simulink model "DeltaWingPlantADRC_FINAL_2018a"  (Simulink 9.1)
settings: Solver=ode45  StartTime=0.0  StopTime=100  MaxStep=0.01  RelTol=1e-3  EnableMultiTasking=on
values from neighbouring files (symbols this model uses):
  beta0 = 0.4    [SA_ACex6_INIT.m]
  betap0 = 0    [SA_ACex6_INIT.m]
  Ta = 0.01    [SA_ACex6_INIT.m]
  um = pi    (= 3.14159265359)    [SA_ACex6_INIT.m]
libraries: simulink x1
settings Model: Creator=Adam  LastModifiedBy=Adam
settings DataIOCC: LimitDataPoints=on  SignalLoggingSaveFormat=ModelDataLogs
settings OptimizationCC: InitFltsAndDblsToZero=on
settings DebuggingCC: SaveWithParameterizedLinksMsg=none  SignalResolutionControl=TryResolveAllWithWarning  SolverPrmCheckMsg=warning  MultiTaskDSMMsg=warning  MultiTaskCondExecSysMsg=none  FcnCallInpInsideContextMsg=warning
settings SFSimCC: SimUseLocalCustomCode=on
settings RTWCC: RTWUseLocalCustomCode=on
settings GRTTargetCC: TargetFcnLib=ansi_tfl_tmw.mat
settings ConfigComp: CovExternalEMLEnable=on

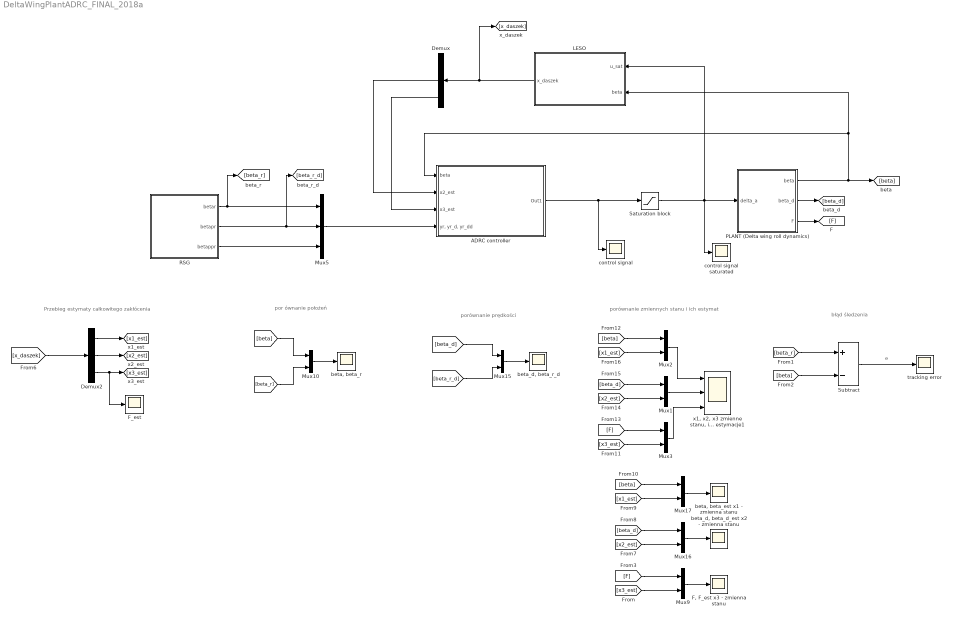
== system DeltaWingPlantADRC_FINAL_2018a ==
  note: Przebieg estymaty całkowitego zakłócenia
  note: błąd śledzenia
  note: e
  note: porównanie prędkości
  note: por ównanie położeń
  note: porównanie zmiennych stanu i ich estymat
  ADRC controller : Subsystem
  Demux : Demux  Outputs=3
  Demux2 : Demux  Outputs=3
  "F, F_est x3 - zmienna stanu" : Scope
  F_est : Scope
  LESO : Subsystem
  Mux{1..3,9..10,15..17} (8 alike) : Mux  Inputs=2
  Mux5 : Mux  Inputs=3
  PLANT (Delta wing roll dynamics) : Subsystem
  RSG : Subsystem
  Saturation block : Saturate  UpperLimit=um  LowerLimit=-um
  Subtract : Sum  Inputs=+-
  "beta, beta_est x1 - zmienna stanu" : Scope
  "beta, beta_r" : Scope
  "beta_d, beta_d_est x2 - zmienna stanu" : Scope
  "beta_d, beta_r_d" : Scope
  control signal : Scope
  control signal saturated : Scope
  tracking error : Scope
  "x1, x2, x3 zmienne stanu, ich estymacje1" : Scope  NumInputPorts=3
  wires:
  RSG/3(betappr) -> Mux5/3
  ADRC controller/1(Out1) -> Saturation block/1, control signal/1
  PLANT (Delta wing roll dynamics)/1(beta) -> [beta], ADRC controller/1(beta), LESO/2(beta)
  Demux/3 -> ADRC controller/3(x3_est)
  Mux5/1 -> ADRC controller/4("yr, yr_d, yr_dd")
  Demux/2 -> ADRC controller/2(x2_est)
  Saturation block/1 -> control signal saturated/1, PLANT (Delta wing roll dynamics)/1(delta_a), LESO/1(u_sat)
  RSG/1(betar) -> [beta_r], Mux5/1
  RSG/2(betapr) -> [beta_r_d], Mux5/2
  [beta_r] -> Subtract/1
  [beta] -> Subtract/2
  Subtract/1 -> tracking error/1
  [F] -> Mux9/1
  Mux9/1 -> "F, F_est x3 - zmienna stanu"/1
  Mux10/1 -> "beta, beta_r"/1
  [x_daszek] -> Demux2/1
  Demux2/1 -> [x1_est]
  Demux2/2 -> [x2_est]
  Demux2/3 -> F_est/1, [x3_est]
  [x3_est] -> Mux9/2
  Mux15/1 -> "beta_d, beta_r_d"/1
  [beta_r_d] -> Mux15/2
  [beta_d] -> Mux15/1
  [beta_d] -> Mux16/1
  [x2_est] -> Mux16/2
  Mux16/1 -> "beta_d, beta_d_est x2 - zmienna stanu"/1
  [beta] -> Mux17/1
  [x1_est] -> Mux17/2
  Mux17/1 -> "beta, beta_est x1 - zmienna stanu"/1
  [beta_r] -> Mux10/2
  [beta] -> Mux10/1
  LESO/1(x_daszek) -> [x_daszek], Demux/1
  PLANT (Delta wing roll dynamics)/2(beta_d) -> [beta_d]
  PLANT (Delta wing roll dynamics)/3(F) -> [F]
  Mux2/1 -> "x1, x2, x3 zmienne stanu, ich estymacje1"/1
  Mux1/1 -> "x1, x2, x3 zmienne stanu, ich estymacje1"/2
  [beta] -> Mux2/1
  [F] -> Mux3/1
  [x3_est] -> Mux3/2
  [x2_est] -> Mux1/2
  [beta_d] -> Mux1/1
  Mux3/1 -> "x1, x2, x3 zmienne stanu, ich estymacje1"/3
  [x1_est] -> Mux2/2

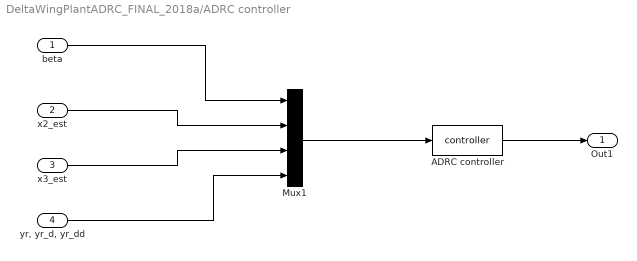
== system DeltaWingPlantADRC_FINAL_2018a/ADRC controller ==
  beta : Inport
  x2_est : Inport  Port=2
  x3_est : Inport  Port=3
  "yr, yr_d, yr_dd" : Inport  Port=4
  ADRC controller : MATLABFcn  MATLABFcn=controller
  Mux1 : Mux
  Out1 : Outport
  wires:
  Mux1/1 -> ADRC controller/1
  ADRC controller/1 -> Out1/1
  beta/1 -> Mux1/1
  x2_est/1 -> Mux1/2
  x3_est/1 -> Mux1/3
  "yr, yr_d, yr_dd"/1 -> Mux1/4

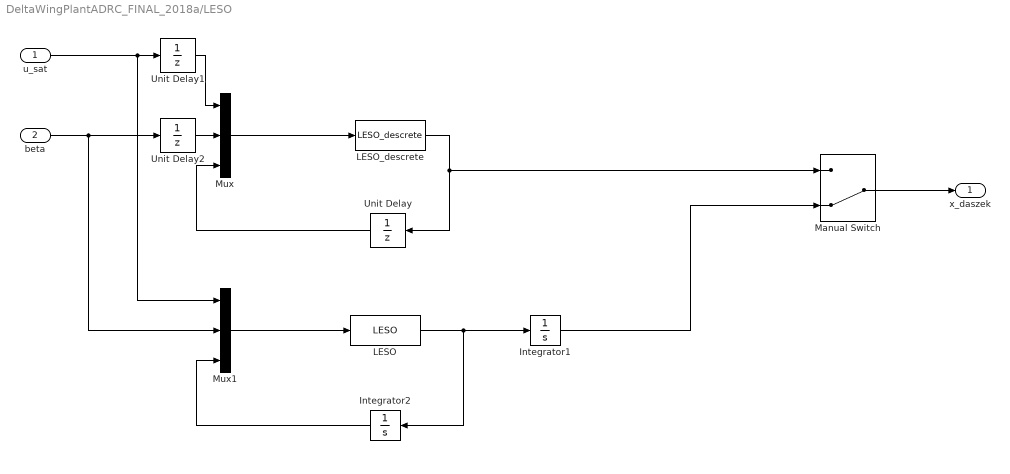
== system DeltaWingPlantADRC_FINAL_2018a/LESO ==
  u_sat : Inport
  beta : Inport  Port=2
  Integrator1 : Integrator  InitialCondition=[0 0 0]
  Integrator2 : Integrator  InitialCondition=[0 0 0]
  LESO : MATLABFcn  MATLABFcn=LESO  OutputDimensions=3
  LESO_descrete : MATLABFcn  MATLABFcn=LESO_descrete  OutputDimensions=3
  Manual Switch : ManualSwitch  CurrentSetting=0
  Mux : Mux  Inputs=3
  Mux1 : Mux  Inputs=3
  Unit Delay : UnitDelay  SampleTime=Ta  HasFrameUpgradeWarning=on
  Unit Delay1 : UnitDelay  SampleTime=Ta  HasFrameUpgradeWarning=on
  Unit Delay2 : UnitDelay  SampleTime=Ta  HasFrameUpgradeWarning=on
  x_daszek : Outport
  wires:
  LESO/1 -> Integrator2/1, Integrator1/1
  Mux/1 -> LESO_descrete/1
  u_sat/1 -> Mux1/1, Unit Delay1/1
  beta/1 -> Mux1/2, Unit Delay2/1
  LESO_descrete/1 -> Unit Delay/1, Manual Switch/1
  Unit Delay/1 -> Mux/3
  Mux1/1 -> LESO/1
  Integrator2/1 -> Mux1/3
  Integrator1/1 -> Manual Switch/2
  Manual Switch/1 -> x_daszek/1
  Unit Delay1/1 -> Mux/1
  Unit Delay2/1 -> Mux/2

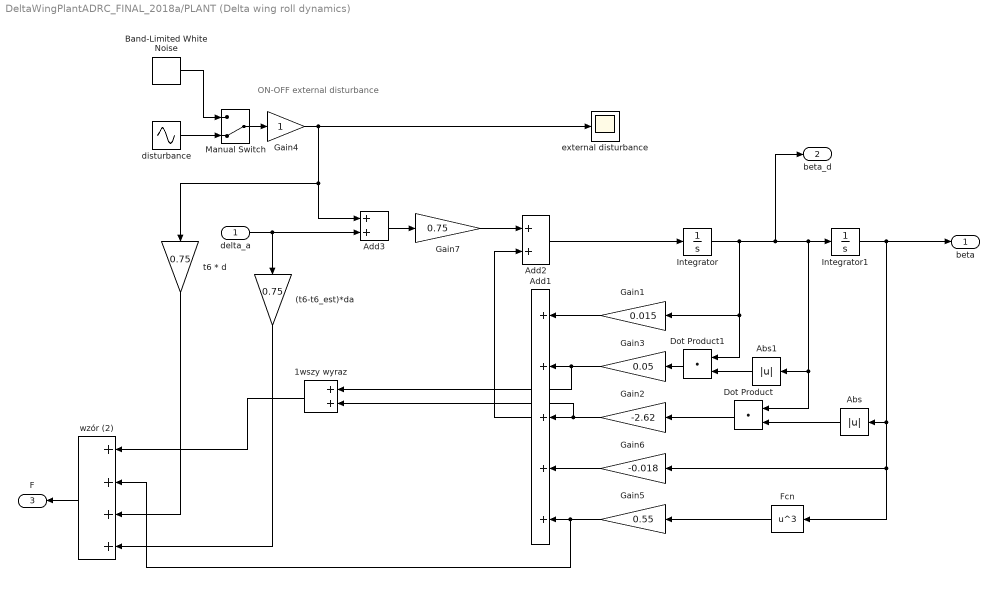
== system DeltaWingPlantADRC_FINAL_2018a/PLANT (Delta wing roll dynamics) ==
  note: ON-OFF external
      | disturbance
  delta_a : Inport
  (t6-t6_est)*da : Gain  Gain=0.75
  1wszy wyraz : Sum
  Abs : Abs
  Abs1 : Abs
  Add1 : Sum  Inputs=+++++
  Add2 : Sum
  Add3 : Sum
  Band-Limited White Noise : simulink/Sources/Band-Limited White Noise  Cov=[0.1*15]  Ts=15  seed=[23341]
  Dot Product : DotProduct  InputSameDT=on  OutDataTypeStr=Inherit: Inherit via internal rule
  Dot Product1 : DotProduct  InputSameDT=on  OutDataTypeStr=Inherit: Inherit via internal rule
  Fcn : Fcn  Expr=u^3
  Gain1 : Gain  Gain=0.015
  Gain2 : Gain  Gain=-2.62
  Gain3 : Gain  Gain=0.05
  Gain4 : Gain
  Gain5 : Gain  Gain=0.55
  Gain6 : Gain  Gain=-0.018
  Gain7 : Gain  Gain=0.75
  Integrator : Integrator  InitialCondition=betap0
  Integrator1 : Integrator  InitialCondition=beta0
  Manual Switch : ManualSwitch  CurrentSetting=0
  disturbance : Sin  Amplitude=1.5  SampleTime=0
  external disturbance : Scope
  t6 * d : Gain  Gain=0.75
  wzór (2) : Sum  Inputs=++++
  beta : Outport
  beta_d : Outport  Port=2
  F : Outport  Port=3
  wires:
  Integrator/1 -> Dot Product1/1, Gain1/1, beta_d/1, Integrator1/1, Dot Product/1, Abs1/1
  Add2/1 -> Integrator/1
  Manual Switch/1 -> Gain4/1
  Band-Limited White Noise/1 -> Manual Switch/1
  disturbance/1 -> Manual Switch/2
  Integrator1/1 -> beta/1, Gain6/1, Fcn/1, Abs/1
  Add1/1 -> Add2/2
  Fcn/1 -> Gain5/1
  Dot Product/1 -> Gain2/1
  Abs/1 -> Dot Product/2
  Abs1/1 -> Dot Product1/2
  Dot Product1/1 -> Gain3/1
  Gain1/1 -> Add1/1
  Gain3/1 -> 1wszy wyraz/1, Add1/2
  Gain2/1 -> 1wszy wyraz/2, Add1/3
  Gain6/1 -> Add1/4
  Gain5/1 -> wzór (2)/2, Add1/5
  Gain4/1 -> external disturbance/1, t6 * d/1, Add3/1
  Add3/1 -> Gain7/1
  delta_a/1 -> Add3/2, (t6-t6_est)*da/1
  Gain7/1 -> Add2/1
  1wszy wyraz/1 -> wzór (2)/1
  t6 * d/1 -> wzór (2)/3
  (t6-t6_est)*da/1 -> wzór (2)/4
  wzór (2)/1 -> F/1

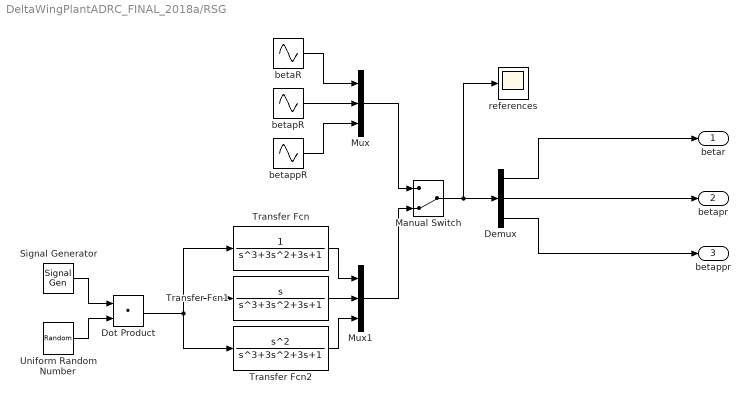
== system DeltaWingPlantADRC_FINAL_2018a/RSG ==
  Demux : Demux  Outputs=3
  Dot Product : DotProduct  InputSameDT=on  OutDataTypeStr=Inherit: Inherit via internal rule
  Manual Switch : ManualSwitch  CurrentSetting=0
  Mux : Mux  Inputs=3
  Mux1 : Mux  Inputs=3
  Signal Generator : SignalGenerator  WaveForm=square  Frequency=0.05
  Transfer Fcn : TransferFcn  Denominator=[1 3 3 1]
  Transfer Fcn1 : TransferFcn  Numerator=[1 0]  Denominator=[1 3 3 1]
  Transfer Fcn2 : TransferFcn  Numerator=[1 0 0]  Denominator=[1 3 3 1]
  Uniform Random Number : UniformRandomNumber  Minimum=-0.8*pi/2  Maximum=0.8*pi/2  SampleTime=10
  betaR : Sin  Frequency=0.5  SampleTime=0
  betapR : Sin  Amplitude=0.5  Frequency=0.5  Phase=pi/2  SampleTime=0
  betappR : Sin  Amplitude=-1*0.5*0.5  Frequency=0.5  SampleTime=0
  references : Scope
  betar : Outport
  betapr : Outport  Port=2
  betappr : Outport  Port=3
  wires:
  betaR/1 -> Mux/1
  betapR/1 -> Mux/2
  betappR/1 -> Mux/3
  Mux/1 -> Manual Switch/1
  Mux1/1 -> Manual Switch/2
  Manual Switch/1 -> Demux/1, references/1
  Demux/2 -> betapr/1
  Demux/1 -> betar/1
  Demux/3 -> betappr/1
  Transfer Fcn/1 -> Mux1/1
  Transfer Fcn1/1 -> Mux1/2
  Transfer Fcn2/1 -> Mux1/3
  Signal Generator/1 -> Dot Product/1
  Uniform Random Number/1 -> Dot Product/2
  Dot Product/1 -> Transfer Fcn1/1, Transfer Fcn/1, Transfer Fcn2/1
